simulink model "obstacleDetection_onoff_VEX"  (R2017a)
settings: Solver=FixedStepAuto  StartTime=0.0  StopTime=inf  FixedStep=Ts  RelTol=1e-3  EnableMultiTasking=on
PreLoadFcn:
  | robotParameters;
values from neighbouring files (symbols this model uses):
  motorIp = [-127 -126 -125 -124 -123 -122 -121 -120 -119 -118 -117 -116 ... (255 elements, 1x255)]    [wheelMotorLUT.mat]
  motorSp = [-13.0232004431 -12.9206555577 -12.8181106723 -12.7155657869 -12.6130209016 -12.5104760162 -12.4079311308 -12.3053862454 -12.20284136 -12.1002964747 -11.9977515893 -11.8952067039 ... (255 elements, 1x255)]    [wheelMotorLUT.mat]
undefined symbols (not defined in the file or in its folder): Ts
libraries: vexarmcortexlib x3, mobileRoboticsTrainingLib x1
settings Model: ExtModeTrigDuration=25  Creator=sseshadr  LastModifiedBy=shiremat
settings OptimizationCC: PassReuseOutputArgsAs=Individual arguments  MaxStackSize=64
settings DebuggingCC: ParameterTunabilityLossMsg=error
settings HardwareCC: ProdBitPerPointer=32  ProdBitPerSizeT=32  ProdBitPerPtrDiffT=32  ProdLargestAtomicInteger=Long  ProdLargestAtomicFloat=Double  ProdWordSize=32  ProdHWDeviceType=ARM Compatible->ARM Cortex
settings SFSimCC: MATLABDynamicMemAlloc=off
settings RTWCC: SystemTargetFile=ert.tlc  HardwareBoard=ARM Cortex-based VEX Microcontroller  TLCOptions="-aInlineSetEventsForThisBaseRateFcn=TLC_FALSE -aSuppressMultiTaskScheduler=TLC_FALSE  -aRateBasedStepFcn=0"  TemplateMakefile=ert_default_tmf  Description=Embedded Coder  GenerateReport=on  Toolchain=GNU Tools for VEX ARM Cortex  IncludeHyperlinkInReport=on  LaunchReport=on  GenerateTraceInfo=on  GenerateTraceReport=on  GenerateTraceReportSl=on  GenerateTraceReportSf=on  GenerateTraceReportEml=on
settings CodeAppCC: ForceParamTrailComments=on  IgnoreCustomStorageClasses=off  OperatorAnnotations=on  SimulinkDataObjDesc=on  SFDataObjDesc=on  MATLABFcnDesc=on  InsertBlockDesc=on  MATLABSourceComments=on

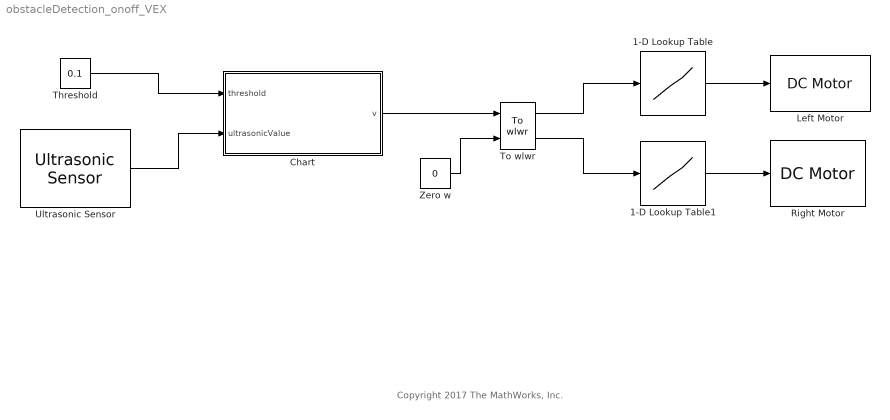
== system obstacleDetection_onoff_VEX ==
  note: Copyright 2017 The MathWorks, Inc.
  1-D Lookup Table : Lookup_n-D  NumberOfTableDimensions=1  BreakpointsForDimension1=motorSp  Table=motorIp  ExtrapMethod=Clip  InternalRulePriority=Speed  RndMeth=Simplest  InputSameDT=on
  1-D Lookup Table1 : Lookup_n-D  NumberOfTableDimensions=1  BreakpointsForDimension1=motorSp  Table=motorIp  ExtrapMethod=Clip  InternalRulePriority=Speed  RndMeth=Simplest  InputSameDT=on
  Chart : Stateflow chart  TreatAsAtomicUnit=on
  Left Motor : vexarmcortexlib/Actuators/DC Motor  motor=10  scaleFactor=1/13.5  SimulationOut=off
      settings: SourceProductName=Simulink Coder Support Package for ARM Cortex-based VEX Microcontroller  SourceProductBaseCode=EC_VEX_MICRO
  Right Motor : vexarmcortexlib/Actuators/DC Motor  motor=1  scaleFactor=1/13.5  SimulationOut=off
      settings: SourceProductName=Simulink Coder Support Package for ARM Cortex-based VEX Microcontroller  SourceProductBaseCode=EC_VEX_MICRO
  Threshold : Constant  Value=0.1
  To wlwr : mobileRoboticsTrainingLib/To wlwr  axleLength=axleLength  wheelR=wheelR
  Ultrasonic Sensor : vexarmcortexlib/Sensors/Ultrasonic Sensor  inputPin=7  outputPin=6  inputPortSim=off  SampleTime=Ts
      settings: SourceProductName=Simulink Coder Support Package for ARM Cortex-based VEX Microcontroller  SourceProductBaseCode=EC_VEX_MICRO
  Zero w : Constant  Value=0
  wires:
  1-D Lookup Table1/1 -> Right Motor/1
  1-D Lookup Table/1 -> Left Motor/1
  To wlwr/1 -> 1-D Lookup Table/1
  To wlwr/2 -> 1-D Lookup Table1/1
  Chart/1(v) -> To wlwr/1
  Zero w/1 -> To wlwr/2
  Ultrasonic Sensor/1 -> Chart/2(ultrasonicValue)
  Threshold/1 -> Chart/1(threshold)

== stateflow chart obstacleDetection_onoff_VEX/Chart ==
  state Go
    entry: v = 0.2;
  state Stop
    entry: v = 0;
  (default) -> Go
  Go -> Stop : [(ultrasonicValue <= threshold) && (ultrasonicValue > 0)]
  Stop -> Go : [ultrasonicValue > threshold]
  data: threshold input; ultrasonicValue input; v output
